simulink model "stm32f4_can_demo"  (Simulink 8.2)
settings: Solver=FixedStepDiscrete  SolverMode=SingleTasking  StartTime=0.0  StopTime=10.0  RelTol=1e-3
PreLoadFcn:
  | waijung.modelPreload; % Required for working with Waijung Blockset. Do not remove.
undefined symbols (not defined in the file): HSEOSC, Link, LQFP176, ST, STM32F417IG
libraries: simulink x10, stm32f4_canbus_lib x5, stm32f4_io_lib x5, stm32f4_device_config_lib x1
CloseFcn:
  | waijung.modelClose; % Required for working with Waijung Blockset. Do not remove.
settings Model: Creator=Krisada  LastModifiedBy=Krisada
settings OptimizationCC: OptimizeModelRefInitCode=on  LifeSpan=1
settings HardwareCC: ProdEndianess=LittleEndian  ProdHWDeviceType=ARM Compatible->Cortex - M4  TargetEndianess=LittleEndian  TargetHWDeviceType=ARM Compatible->Cortex - M4
settings RTWCC: SystemTargetFile=stm32f4.tlc  GenerateMakefile=off  TemplateMakefile=ert_default_tmf  Description=STM32F4 Target  ProcessScript=stm32f4_make_rtw_hook
settings CodeAppCC: IgnoreCustomStorageClasses=off  CustomSymbolStrType=$N$R$M  InternalIdentifier=Classic
settings STFCustomTargetCC: CodeReplacementLibrary=ANSI_C  ModelReferenceCompliant=off  CombineOutputUpdateFcns=on  ERTCustomFileBanners=on  SupportContinuousTime=off  SupportNonInlinedSFcns=off  MATLABClassNameForMDSCustomization=Simulink.SoftwareTarget.ERTCustomization  GRTInterface=off  SystemTargetFile=stm32f4.tlc
settings ERTTargetCC: CodeReplacementLibrary=ANSI_C  MultiwordLength=2048  ModelReferenceCompliant=off  ParMdlRefBuildCompliant=off  CompOptLevelCompliant=off  ConcurrentExecutionCompliant=off  ERTFirstTimeCompliant=off  ModelStepFunctionPrototypeControlCompliant=off  CPPClassGenCompliant=off  ExtModeMexFile=noextcomm  InlinedParameterPlacement=NonHierarchical  ERTSrcFileBannerTemplate=stm32f4_code_template.cgt  ERTHdrFileBannerTemplate=stm32f4_code_template.cgt  ERTDataSrcFileTemplate=stm32f4_code_template.cgt  ERTDataHdrFileTemplate=stm32f4_code_template.cgt  ERTCustomFileTemplate=stm32f4_file_process.tlc  ConvertIfToSwitch=off  SuppressUnreachableDefaultCases=off

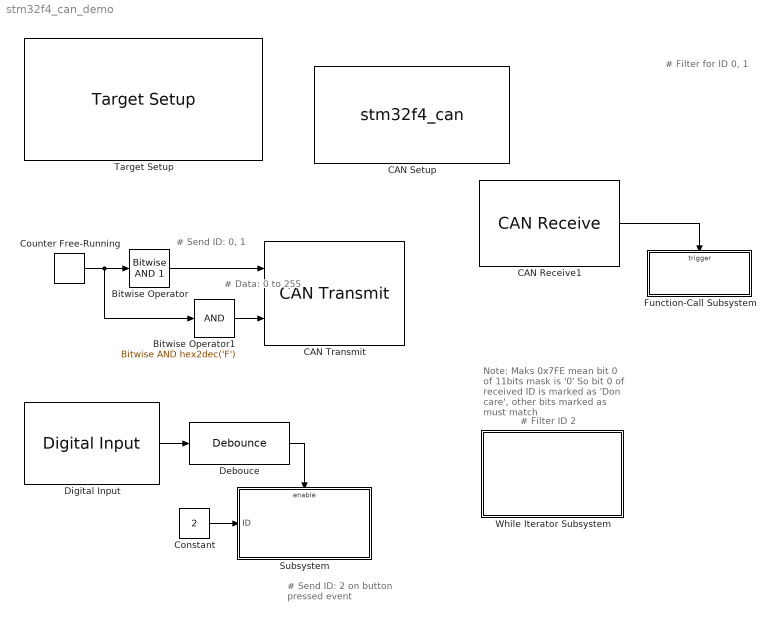
== system stm32f4_can_demo ==
  note: # Send ID: 0, 1
  note: # Data: 0 to 255
  note: # Send ID: 2 on button pressed event
  note: # Filter for ID 0, 1
  note: Note: Maks 0x7FE mean bit 0 of 11bits mask is '0'
      | So bit 0 of received ID is marked as 'Don care',
      | other bits marked as must match
  note: # Filter ID 2
  Bitwise Operator : simulink/Logic and Bit Operations/Bitwise Operator  logicop=AND  UseBitMask=on  BitMask=1  BitMaskRealWorld=Stored Integer
  Bitwise Operator1 : simulink/Logic and Bit Operations/Bitwise Operator  logicop=AND  UseBitMask=on  BitMask=hex2dec('F')  BitMaskRealWorld=Stored Integer
  CAN Receive1 : stm32f4_canbus_lib/CAN Receive  conf=Rx  canmodule=1  idtype=Standard  filtertype=Mask  id=0  idmask=hex2dec('7FE')  enableisr=on  usedlc=off  datatype=single  data0type=int8  data1type=int32  data2type=uint16  data3type=Not used  data4type=Not used  data5type=Not used  data6type=Not used  data7type=Not used  buffersize=8  sampletime=-1  sampletimestr=0.01  blockid=CANReceive1  inputarray=[]  inputlabelarray={}  outputarray=[7]  outputlabelarray={'Call ISR' }  compat=0  confstr="[\"Standard\",\"Mask\",\"0\",\"2046\",\"off\",\"int8\",\"int32\",\"uint16\",\"Not used\",\"Not used\",\"Not used\",\"Not used\",\"Not used\",\"8\",\"0\",\"0\",\"FFC0\",\"4\"]"
  CAN Setup : S-Function  FunctionName=stm32f4_can  Parameters=conf,canmodule,0,inputarray,outputarray,'','',confstr,sampletime,sampletimestr,blockid  EnableBusSupport=off  mask(stm32f4_can){conf=Setup, canmodule=1, advance=off, bitrate_select=125000, sjw=1tq, bs1=14tq, bs2=6tq, timingconf=Prescaler, brp=16, bitrate=125000, tq=3.8095e-07, remaptxpin=B9, remaprxpin=B8, sampletime=-1, sampletimestr=0.01, blockid=CANSetup, inputarray=[], inputlabelarray={}, outputarray=[], outputlabelarray={}, compat=0, confstr=["125000","16","B","9","B","8","1tq","14tq","6tq","ENABLE"], presc=16, txportstr=B, txpinstr=9, rxportstr=B, rxpinstr=8, lastmodule=1}
      mask prompts: conf "Configuration"; canmodule "CAN Module"; advance "Advance configuration"; bitrate_select "Baud rate (bps)"; sjw "Resync Jump Width (SJW)"; bs1 "Bit segment 1 (BS1) + PROP_SEG"; bs2 "Bit segment 2 (BS2)"; timingconf "Adjust"; brp "Baud rate prescaler (BRP)"; bitrate "Baud rate (bps)"; tq "Time Quantum (Second), tq"; remaptxpin "CAN Tx pin"; remaprxpin "CAN Rx pin"; sampletime "Sample time (sec)"; sampletimestr "Compiled sample time (sec) in string"; inputarray "Input port"; inputlabelarray "Input port label"; outputarray "Output port"; outputlabelarray "Output port label"; compat "Compatibility (Reserved for future use)"; confstr "Configuration String"; presc "Prescale"; txportstr "Tx port string"; txpinstr "Tx pin string"; rxportstr "Rx port string"; rxpinstr "Rx pin string"; lastmodule "Last module selected"
      mask help: This block setups CAN Module.
      mask init:
      | stm32f4_can_callback('init');
      mask Help: web(fullfile(waijungdocroot,'stm32f4_can_setup.htm'), '-browser')
      mask TypeOptions conf: Setup
      mask TypeOptions canmodule: 1 | 2
      mask Callback canmodule: stm32f4_can_callback('canmodule');
      mask Callback advance: stm32f4_can_callback('advance');
      mask TypeOptions bitrate_select: 125000 | 250000 | 500000 | 1000000
      mask Callback bitrate_select: stm32f4_can_callback('bitrate_select');
      mask TypeOptions sjw: 1tq | 2tq | 3tq | 4tq
      mask TypeOptions bs1: 1tq | 2tq | 3tq | 4tq | 5tq | 6tq | 7tq | 8tq | 9tq | 10tq | 11tq | 12tq | 13tq | 14tq | 15tq | 16tq
      mask Callback bs1: stm32f4_can_callback('timingconf');
      mask TypeOptions bs2: 1tq | 2tq | 3tq | 4tq | 5tq | 6tq | 7tq | 8tq
      mask Callback bs2: stm32f4_can_callback('timingconf');
      mask TypeOptions timingconf: Prescaler | Baudrate
      mask Callback timingconf: stm32f4_can_callback('timingconf');
      mask Callback brp: stm32f4_can_callback('timingconf');
      mask Callback bitrate: stm32f4_can_callback('timingconf');
      mask TypeOptions remaptxpin: Not used | A12 | B9 | D1 | H13
      mask Callback remaptxpin: stm32f4_can_callback('remaptxpin');
      mask TypeOptions remaprxpin: Not used | A11 | B8 | D0 | I9
      mask Callback remaprxpin: stm32f4_can_callback('remaprxpin');
      mask Callback sampletime: stm32f4_can_callback('sampletime');
      mask Callback sampletimestr: stm32f4_can_callback('sampletimestr');
      mask Callback blockid: stm32f4_can_callback('blockid');
      mask Display: text(0.5, 0.5, 'CAN1_Setup\nSpeed (bps): 125000\nTx/Rx pin: B9/B8','ver','middle','hor','center');
  CAN Transmit : stm32f4_canbus_lib/CAN Transmit  conf=Tx  canmodule=1  transfer=Blocking  timeout=0.001  idtype=Standard  specificid=off  id=0  specificdlc=on  dlc=4  enablestatus=off  datatype=uint32  data0type=uint32  data1type=Not used  data2type=Not used  data3type=Not used  data4type=Not used  data5type=Not used  data6type=Not used  data7type=Not used  inputarray=[ -1, 7]  inputlabelarray={ 'ID', 'D0 (uint32)' }  outputarray=[]  outputlabelarray={}  sampletime=-1  sampletimestr=0.01  blockid=CANTransmit  compat=0  confstr="[\"Blocking\",\"0.001\",\"Standard\",\"off\",\"0\",\"on\",\"4\",\"off\",\"uint32\",\"Not used\",\"Not used\",\"Not used\",\"Not used\",\"Not used\",\"Not used\",\"Not used\"]"
  Constant : Constant  Value=2  SampleTime=-1
  Counter Free-Running : simulink/Sources/Counter Free-Running  NumBits=32  tsamp=0.01
  Debouce : stm32f4_io_lib/Debounce  mode=Single Pulse  prescale=4  debounce=4
  Digital Input : stm32f4_io_lib/Digital Input  port=A  speed=100  porttype=None  porttypestr=NOPULL  use_pin0=on  use_pin1=off  use_pin2=off  use_pin3=off  use_pin4=off  use_pin5=off  use_pin6=off  use_pin7=off  use_pin8=off  use_pin9=off  use_pin10=off  use_pin11=off  use_pin12=off  use_pin13=off  use_pin14=off  use_pin15=off  pinstr=GPIO_Pin_0  usedpinarray="[1  0  0  0  0  0  0  0  0  0  0  0  0  0  0  0]"  bitbandingstr="#define DigitalInput_A0 Peripheral_BB(GPIOA->IDR, 0)  /* Output pin */"  sampletime=0.01  sampletimestr=0.01  blockid=DigitalInput  enablecustomportlabel=off  glabalinit=off  cinputportlabel=In1, In2  coutputportlabel=Out1, Out2
  Function-Call Subsystem : Subsystem  TreatAsAtomicUnit=on
  Subsystem : Subsystem
  Target Setup : stm32f4_device_config_lib/Target Setup  Priority=100  compiler=GNU ARM  previous_compiler=GNU ARM  mcu=STM32F417IG (LQFP176)  mcustr=STM32F417IG  clockconfig=HSEOSC-8MHz  system_stm32f4xx_c_path=F:\trunk\targets\stm32f4_target\stm32f4\utils\system_stm32f4xx_default\STM32F40_41xxx\hseosc8mhz  showmemoryconfiguration=off  stacksize=0x2000  heapsize=0x2000  enableautocompiledownload=on  fullchiperase=off  programmerinterface=ST-Link  editctrlstr=on  compilercontrolstr=$(patsubst %, -I%, .) -mcpu=cortex-m4 -mthumb -mthumb-interwork -mfloat-abi=hard -mfpu=fpv4-sp-d16 -ffast-math -Wall -Wextra -Ofast  assemblercontrolstr=$(patsubst %, -I%, .) -mcpu=cortex-m4 -mthumb -mthumb-interwork -mfloat-abi=hard -mfpu=fpv4-sp-d16 -ffast-math -Wall -Wextra -Ofast -Wa,-amhls=$(<:.s=.lst) -D__STACK_SIZE=$(STACK_SIZE) -D__HEAP_SIZE=$(HEAP_SIZE)  linkercontrolstr=-T$(LD_SCRIPT) -g -Wl,-Map=$(MAP),--cref,--no-warn-mismatch -mcpu=cortex-m4 -mthumb -mthumb-interwork -mfloat-abi=hard -mfpu=fpv4-sp-d16 -specs=nosys.specs  runafterdownload=on  execprofile=None  profileruart=3  profilerbaud=500000  profilertxpin=D8  profilerinitstr=0.01,168000000,1680000,500000,0  manualsetsampletime=off  sampletime=0.01  blockid=TargetSetup  systickreloadvalue=1680000  hseval=8000000  lastprofileruart=3  hclk=168000000  flashorigin=0x8000000  flashlength=1024k  ramorigin=0x20000000  ramlength=128k  useextram=off
  While Iterator Subsystem : Subsystem  TreatAsAtomicUnit=on
  wires:
  Counter Free-Running/1 -> Bitwise Operator/1, Bitwise Operator1/1
  Bitwise Operator/1 -> CAN Transmit/1
  Bitwise Operator1/1 -> CAN Transmit/2
  Digital Input/1 -> Debouce/1
  Constant/1 -> Subsystem/1(ID)
  Debouce/1 -> Subsystem/Enable
  CAN Receive1/1 -> Function-Call Subsystem/Trigger

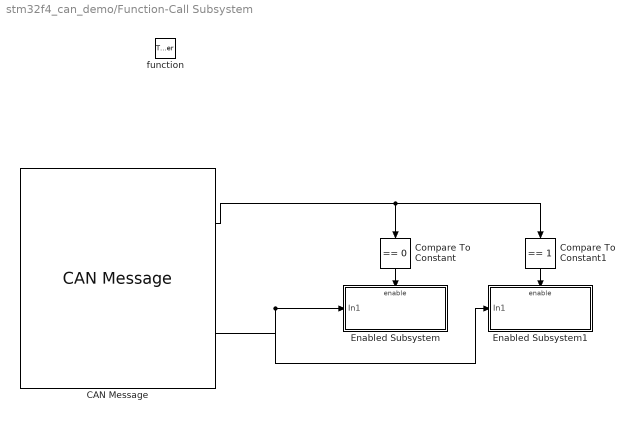
== system stm32f4_can_demo/Function-Call Subsystem ==
  function : TriggerPort  TriggerType=function-call
  CAN Message : stm32f4_canbus_lib/CAN Message  conf=Msg  canmodule=1  usedlc=off  datatype=uint32  data0type=uint32  data1type=Not used  data2type=Not used  data3type=Not used  data4type=Not used  data5type=Not used  data6type=Not used  data7type=Not used  sampletime=-1  sampletimestr=-1  blockid=FunctionCallSubsystemCANMessage  inputarray=[]  inputlabelarray={}  outputarray=[ 7, 7]  outputlabelarray={'ID', 'D0 (uint32)' }  compat=0  confstr="[\"off\",\"uint32\",\"Not used\",\"Not used\",\"Not used\",\"Not used\",\"Not used\",\"Not used\",\"Not used\"]"
  Compare To Constant : simulink/Logic and Bit Operations/Compare To Constant  relop===  const=0  OutDataTypeStr=uint8  ZeroCross=off
  Compare To Constant1 : simulink/Logic and Bit Operations/Compare To Constant  relop===  const=1  OutDataTypeStr=uint8  ZeroCross=off
  Enabled Subsystem : Subsystem  TreatAsAtomicUnit=on
  Enabled Subsystem1 : Subsystem  TreatAsAtomicUnit=on
  wires:
  Compare To Constant/1 -> Enabled Subsystem/Enable
  CAN Message/1 -> Compare To Constant/1, Compare To Constant1/1
  Compare To Constant1/1 -> Enabled Subsystem1/Enable
  CAN Message/2 -> Enabled Subsystem/1(In1), Enabled Subsystem1/1(In1)

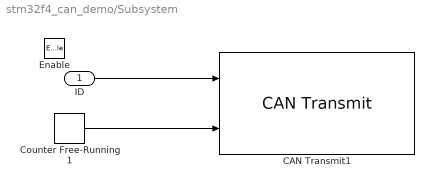
== system stm32f4_can_demo/Subsystem ==
  ID : Inport
  Enable : EnablePort  PropagateVarSize=During execution
  CAN Transmit1 : stm32f4_canbus_lib/CAN Transmit  conf=Tx  canmodule=1  transfer=Blocking  timeout=0.001  idtype=Standard  specificid=off  id=2  specificdlc=on  dlc=4  enablestatus=off  datatype=uint32  data0type=uint32  data1type=Not used  data2type=Not used  data3type=Not used  data4type=Not used  data5type=Not used  data6type=Not used  data7type=Not used  inputarray=[ -1, 7]  inputlabelarray={ 'ID', 'D0 (uint32)' }  outputarray=[]  outputlabelarray={}  sampletime=-1  sampletimestr=0.01  blockid=SubsystemCANTransmit1  compat=0  confstr="[\"Blocking\",\"0.001\",\"Standard\",\"off\",\"2\",\"on\",\"4\",\"off\",\"uint32\",\"Not used\",\"Not used\",\"Not used\",\"Not used\",\"Not used\",\"Not used\",\"Not used\"]"
  Counter Free-Running1 : simulink/Sources/Counter Free-Running  NumBits=32  tsamp=-1
  wires:
  Counter Free-Running1/1 -> CAN Transmit1/2
  ID/1 -> CAN Transmit1/1

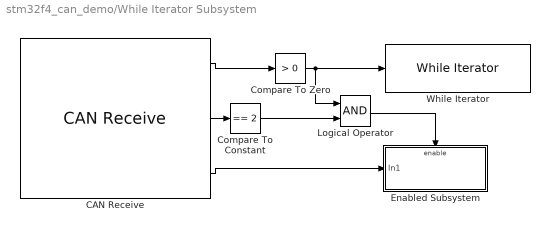
== system stm32f4_can_demo/While Iterator Subsystem ==
  CAN Receive : stm32f4_canbus_lib/CAN Receive  conf=Rx  canmodule=1  idtype=Standard  filtertype=Specific  id=2  idmask=0  enableisr=off  usedlc=off  datatype=uint32  data0type=uint32  data1type=Not used  data2type=Not used  data3type=Not used  data4type=Not used  data5type=Not used  data6type=Not used  data7type=Not used  buffersize=8  sampletime=-1  sampletimestr=-1  blockid=WhileIteratorSubsystemCANReceive  inputarray=[]  inputlabelarray={}  outputarray=[ 5, 7, 7]  outputlabelarray={ 'Msg Pending','ID', 'D0 (uint32)' }  compat=0  confstr="[\"Standard\",\"Specific\",\"2\",\"0\",\"off\",\"uint32\",\"Not used\",\"Not used\",\"Not used\",\"Not used\",\"Not used\",\"Not used\",\"Not used\",\"8\",\"40\",\"0\",\"FFE0\",\"4\"]"
  Compare To Constant : simulink/Logic and Bit Operations/Compare To Constant  relop===  const=2  OutDataTypeStr=uint8  ZeroCross=off
  Compare To Zero : simulink/Logic and Bit Operations/Compare To Zero  relop=>  OutDataTypeStr=uint8  ZeroCross=off
  Enabled Subsystem : Subsystem  TreatAsAtomicUnit=on
  Logical Operator : Logic  AllPortsSameDT=off  OutDataTypeStr=boolean
  While Iterator : WhileIterator  WhileBlockType=do-while
  wires:
  CAN Receive/1 -> Compare To Zero/1
  Compare To Zero/1 -> While Iterator/1, Logical Operator/1
  CAN Receive/2 -> Compare To Constant/1
  Compare To Constant/1 -> Logical Operator/2
  Logical Operator/1 -> Enabled Subsystem/Enable
  CAN Receive/3 -> Enabled Subsystem/1(In1)

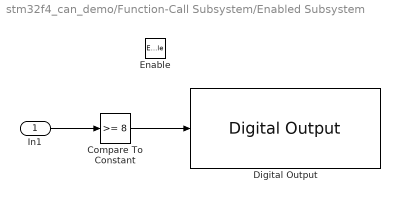
== system stm32f4_can_demo/Function-Call Subsystem/Enabled Subsystem ==
  In1 : Inport
  Enable : EnablePort  PropagateVarSize=During execution
  Compare To Constant : simulink/Logic and Bit Operations/Compare To Constant  relop=>=  const=8  OutDataTypeStr=uint8  ZeroCross=off
  Digital Output : stm32f4_io_lib/Digital Output  use_bitband=on  port=D  speed=100  porttype=Push Pull  porttypestr=PP  use_pin0=off  use_pin1=off  use_pin2=off  use_pin3=off  use_pin4=off  use_pin5=off  use_pin6=off  use_pin7=off  use_pin8=off  use_pin9=off  use_pin10=off  use_pin11=off  use_pin12=on  use_pin13=off  use_pin14=off  use_pin15=off  pinstr=GPIO_Pin_12  usedpinarray="[0  0  0  0  0  0  0  0  0  0  0  0  1  0  0  0]"  bitbandingstr="#define FunctionCallSubsystemEnabledSubsystemDigitalOutput_D12 Peripheral_BB(GPIOD->ODR, 12)  /* Output pin */"  sampletime=-1  sampletimestr=-1  blockid=FunctionCallSubsystemEnabledSubsystemDigitalOutput  enablecustomportlabel=off  globalinit=off  cinputportlabel=In1, In2  coutputportlabel=0
  wires:
  In1/1 -> Compare To Constant/1
  Compare To Constant/1 -> Digital Output/1

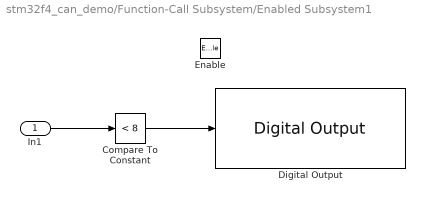
== system stm32f4_can_demo/Function-Call Subsystem/Enabled Subsystem1 ==
  In1 : Inport
  Enable : EnablePort  PropagateVarSize=During execution
  Compare To Constant : simulink/Logic and Bit Operations/Compare To Constant  relop=<  const=8  OutDataTypeStr=uint8  ZeroCross=off
  Digital Output : stm32f4_io_lib/Digital Output  use_bitband=on  port=D  speed=100  porttype=Push Pull  porttypestr=PP  use_pin0=off  use_pin1=off  use_pin2=off  use_pin3=off  use_pin4=off  use_pin5=off  use_pin6=off  use_pin7=off  use_pin8=off  use_pin9=off  use_pin10=off  use_pin11=off  use_pin12=off  use_pin13=on  use_pin14=off  use_pin15=off  pinstr=GPIO_Pin_13  usedpinarray="[0  0  0  0  0  0  0  0  0  0  0  0  0  1  0  0]"  bitbandingstr="#define FunctionCallSubsystemEnabledSubsystem1DigitalOutput_D13 Peripheral_BB(GPIOD->ODR, 13)  /* Output pin */"  sampletime=-1  sampletimestr=-1  blockid=FunctionCallSubsystemEnabledSubsystem1DigitalOutput  enablecustomportlabel=off  globalinit=off  cinputportlabel=In1, In2  coutputportlabel=0
  wires:
  In1/1 -> Compare To Constant/1
  Compare To Constant/1 -> Digital Output/1

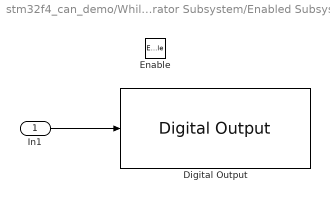
== system stm32f4_can_demo/While Iterator Subsystem/Enabled Subsystem ==
  In1 : Inport
  Enable : EnablePort  PropagateVarSize=During execution
  Digital Output : stm32f4_io_lib/Digital Output  use_bitband=on  port=D  speed=100  porttype=Push Pull  porttypestr=PP  use_pin0=off  use_pin1=off  use_pin2=off  use_pin3=off  use_pin4=off  use_pin5=off  use_pin6=off  use_pin7=off  use_pin8=off  use_pin9=off  use_pin10=off  use_pin11=off  use_pin12=off  use_pin13=off  use_pin14=on  use_pin15=off  pinstr=GPIO_Pin_14  usedpinarray="[0  0  0  0  0  0  0  0  0  0  0  0  0  0  1  0]"  bitbandingstr="#define WhileIteratorSubsystemEnabledSubsystemDigitalOutput_D14 Peripheral_BB(GPIOD->ODR, 14)  /* Output pin */"  sampletime=-1  sampletimestr=-1  blockid=WhileIteratorSubsystemEnabledSubsystemDigitalOutput  enablecustomportlabel=off  globalinit=off  cinputportlabel=In1, In2  coutputportlabel=0
  wires:
  In1/1 -> Digital Output/1
